simulink library "MPC_Controllers"  (R2016b)
settings: Solver=VariableStepAuto  StartTime=0.0  StopTime=10.0  RelTol=1e-3
undefined symbols (not defined in the file or in its folder): nu, ny
settings Model: Creator=asierzubizarreta  LastModifiedBy=asierzubizarreta

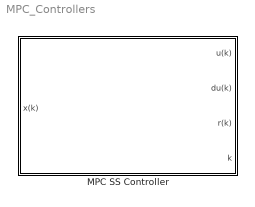
== system MPC_Controllers ==
  MPC SS Controller : Subsystem  InitFcn=|  TreatAsAtomicUnit=on
      | [parameters, Ref,Td]=Initialization_MPC_SS; 
      | [nx,nu]=size(parameters.B);
      | [ny,nx]=size(parameters.C);
      mask DialogControl DescGroupVar Prompt: MPC Controller
      mask Display:
      | fprintf('MPC SS Control\n\n\n');
      | 
      | 
      | port_label('output',1,'u(k)');
      | port_label('output',2,'du(k)');
      | port_label('output',3,'r(k)');
      | port_label('output',4,'k');
      | port_label('input',1,'x(k)');

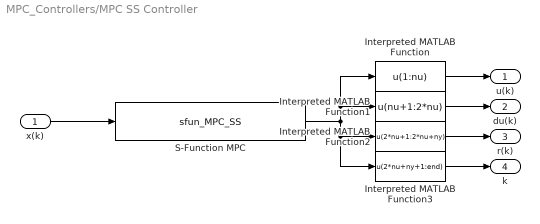
== system MPC_Controllers/MPC SS Controller ==
  x(k) : Inport
  Interpreted MATLAB Function : MATLABFcn  MATLABFcn=u(1:nu)
  Interpreted MATLAB Function1 : MATLABFcn  MATLABFcn=u(nu+1:2*nu)
  Interpreted MATLAB Function2 : MATLABFcn  MATLABFcn=u(2*nu+1:2*nu+ny)
  Interpreted MATLAB Function3 : MATLABFcn  MATLABFcn=u(2*nu+ny+1:end)
  S-Function MPC : S-Function  FunctionName=sfun_MPC_SS  SFunctionModules=s  SFunctionDeploymentMode=off  EnableBusSupport=off
  u(k) : Outport
  du(k) : Outport  Port=2
  r(k) : Outport  Port=3
  k : Outport  Port=4
  wires:
  Interpreted MATLAB Function/1 -> u(k)/1
  Interpreted MATLAB Function1/1 -> du(k)/1
  Interpreted MATLAB Function2/1 -> r(k)/1
  Interpreted MATLAB Function3/1 -> k/1
  x(k)/1 -> S-Function MPC/1
  S-Function MPC/1 -> Interpreted MATLAB Function1/1, Interpreted MATLAB Function/1, Interpreted MATLAB Function3/1, Interpreted MATLAB Function2/1
